simulink model "main"  (R2022b)
settings: Solver=VariableStepAuto  StartTime=0.0  StopTime=inf  RelTol=1e-3
settings Model: Creator=PSSENL  LastModifiedBy=rhdej
settings DebuggingCC: UnderSpecifiedDimensionMsg=warning

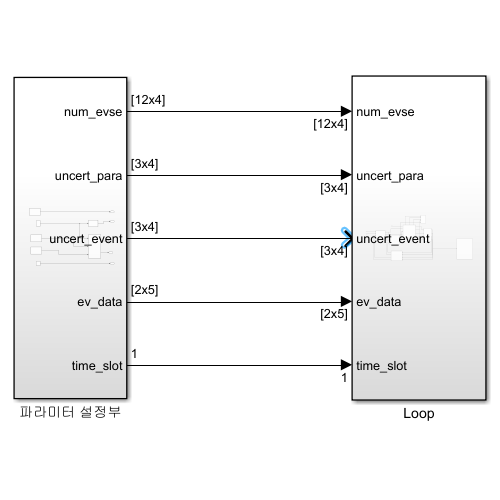
[thumbnail: Simulink's stored preview of the top-level diagram]
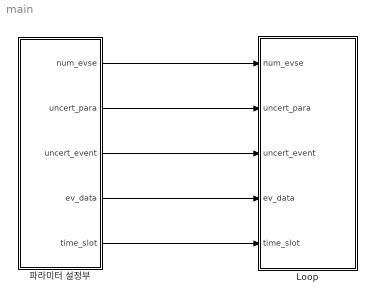
== system main ==
  Loop : Subsystem
  파라미터 설정부 : Subsystem
  wires:
  파라미터 설정부/1(num_evse) -> Loop/1(num_evse)
  파라미터 설정부/4(ev_data) -> Loop/4(ev_data)
  파라미터 설정부/5(time_slot) -> Loop/5(time_slot)
  파라미터 설정부/2(uncert_para) -> Loop/2(uncert_para)
  파라미터 설정부/3(uncert_event) -> Loop/3(uncert_event)

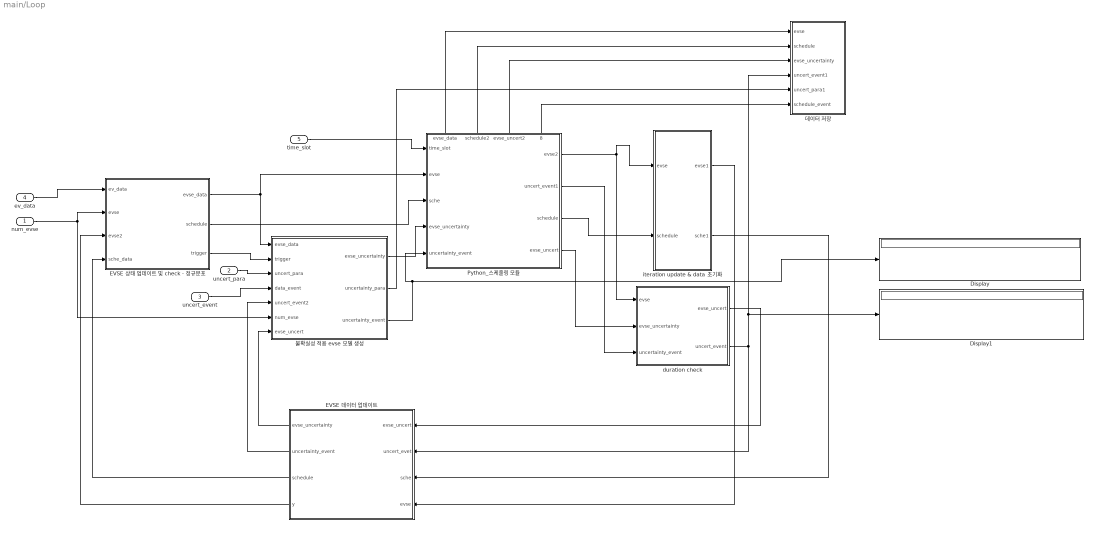
== system main/Loop ==
  num_evse : Inport
  uncert_para : Inport  Port=2
  uncert_event : Inport  Port=3
  ev_data : Inport  Port=4
  time_slot : Inport  Port=5
  Display : Display
  Display1 : Display
  EVSE 데이터 업데이트 : Subsystem
  EVSE 상태 업데이트 및 check - 정규분포 : Subsystem  TreatAsAtomicUnit=on
      settings: MinAlgLoopOccurrences=on
  Python_스케줄링 모듈 : Subsystem  TreatAsAtomicUnit=on
      settings: MinAlgLoopOccurrences=on  PortSchema="{\"entries\":[{\"content\":{\"sides\":[{\"content\":{\"connectorIds\":[\"In1\",\"In2\",\"In3\",\"In4\",\"In5\"]},\"type\":\"ConnectorPlacement.EquallySpacedRectSide\",\"uuid\":\"108a50dd-ff78-47a2-96bb-1485fa352ef4\"},{\"content\":{\"connectorIds\":[\"Out1\",\"Out2\",\"Out3\",\"Out4\"],\"side\":\"RIGHT\"},\"type\":\"ConnectorPlacement.EquallySpacedRectSide\",\"uuid\":\"7c56c117-e709-4297-be3e-b9108604eb1e\"},{\"content\":{\"connectorIds\":[\"Out5\",\"Out6\",\"Out7\",\"Out8\"],\"side\":\"TOP\"},\"type\":\"ConnectorPlacement.EquallySpacedRectSide\",\"uuid\":\"1739f009-047f-4f60-ac68-86188e95dc24\"}]},\"type\":\"ConnectorPlacement.EquallySpacedConnector\",\"uuid\":\"a87990c0-fd82-4870-9496-759f08e65f9c\"}],\"packageUris\":[\"http://schema.mathworks.com/mf0/Connector/R2020b\"],\"version\":\"1.0\"}"
  duration check : MATLAB Function  TreatAsAtomicUnit=on
  iteration update & data 초기화 : MATLAB Function  TreatAsAtomicUnit=on
  데이터 저장 : Subsystem  TreatAsAtomicUnit=on
      settings: MinAlgLoopOccurrences=on
  불확실성 적용 evse 모델 생성 : Subsystem
  wires:
  EVSE 상태 업데이트 및 check - 정규분포/1(evse_data) -> 불확실성 적용 evse 모델 생성/1(evse_data), Python_스케줄링 모듈/2(evse)
  ev_data/1 -> EVSE 상태 업데이트 및 check - 정규분포/1(ev_data)
  iteration update & data 초기화/1(evse1) -> EVSE 데이터 업데이트/4(evse)
  iteration update & data 초기화/2(sche1) -> EVSE 데이터 업데이트/3(sche)
  num_evse/1 -> 불확실성 적용 evse 모델 생성/6(num_evse), EVSE 상태 업데이트 및 check - 정규분포/2(evse)
  EVSE 데이터 업데이트/4(y) -> EVSE 상태 업데이트 및 check - 정규분포/3(evse2)
  EVSE 상태 업데이트 및 check - 정규분포/2(schedule) -> Python_스케줄링 모듈/3(sche)
  Python_스케줄링 모듈/1(evse2) -> iteration update & data 초기화/1(evse), duration check/1(evse)
  Python_스케줄링 모듈/3(schedule) -> iteration update & data 초기화/2(schedule)
  time_slot/1 -> Python_스케줄링 모듈/1(time_slot)
  Python_스케줄링 모듈/5(evse_data) -> 데이터 저장/1(evse)
  Python_스케줄링 모듈/6(schedule2) -> 데이터 저장/2(schedule)
  EVSE 데이터 업데이트/3(schedule) -> EVSE 상태 업데이트 및 check - 정규분포/4(sche_data)
  uncert_para/1 -> 불확실성 적용 evse 모델 생성/3(uncert_para)
  uncert_event/1 -> 불확실성 적용 evse 모델 생성/4(data_event)
  EVSE 상태 업데이트 및 check - 정규분포/3(trigger) -> 불확실성 적용 evse 모델 생성/2(trigger)
  불확실성 적용 evse 모델 생성/1(evse_uncertainty) -> Python_스케줄링 모듈/4(evse_uncertainty)
  불확실성 적용 evse 모델 생성/3(uncertainty_event) -> Python_스케줄링 모듈/5(uncertainty_event), Display/1
  duration check/2(uncert_event) -> EVSE 데이터 업데이트/2(uncert_evet), 데이터 저장/4(uncert_event1), Display1/1
  duration check/1(evse_uncert) -> EVSE 데이터 업데이트/1(evse_uncert)
  Python_스케줄링 모듈/4(evse_uncert) -> duration check/2(evse_uncertainty)
  EVSE 데이터 업데이트/1(evse_uncertainty) -> 불확실성 적용 evse 모델 생성/7(evse_uncert)
  Python_스케줄링 모듈/7(evse_uncert2) -> 데이터 저장/3(evse_uncertainty)
  Python_스케줄링 모듈/2(uncert_event1) -> duration check/3(uncertainty_event)
  불확실성 적용 evse 모델 생성/2(uncertainty_para) -> 데이터 저장/5(uncert_para1)
  EVSE 데이터 업데이트/2(uncertainty_event) -> 불확실성 적용 evse 모델 생성/5(uncert_event2)
  Python_스케줄링 모듈/8(schedule_event) -> 데이터 저장/6(schedule_event)

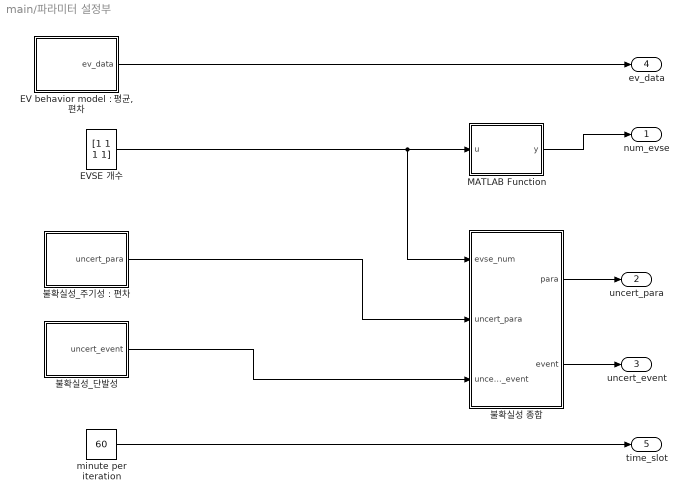
== system main/파라미터 설정부 ==
  "EV behavior model : 평균, 편차" : Subsystem
  EVSE 개수 : Constant  Value=[1 1 1 1]
  MATLAB Function : MATLAB Function  TreatAsAtomicUnit=on
  minute per iteration : Constant  Value=60
  불확실성 종합 : MATLAB Function  TreatAsAtomicUnit=on
  불확실성_단발성 : Subsystem
  "불확실성_주기성 : 편차" : Subsystem
  num_evse : Outport
  uncert_para : Outport  Port=2
  uncert_event : Outport  Port=3
  ev_data : Outport  Port=4
  time_slot : Outport  Port=5
  wires:
  EVSE 개수/1 -> 불확실성 종합/1(evse_num), MATLAB Function/1(u)
  MATLAB Function/1(y) -> num_evse/1
  "EV behavior model : 평균, 편차"/1(ev_data) -> ev_data/1
  minute per iteration/1 -> time_slot/1
  불확실성_단발성/1(uncert_event) -> 불확실성 종합/3(uncert_event)
  "불확실성_주기성 : 편차"/1(uncert_para) -> 불확실성 종합/2(uncert_para)
  불확실성 종합/1(para) -> uncert_para/1
  불확실성 종합/2(event) -> uncert_event/1

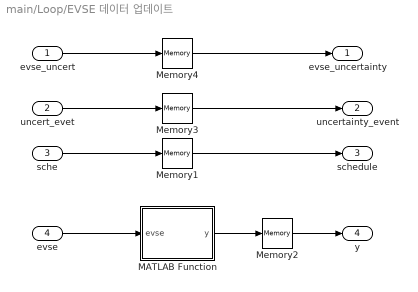
== system main/Loop/EVSE 데이터 업데이트 ==
  evse_uncert : Inport
  uncert_evet : Inport  Port=2
  sche : Inport  Port=3
  evse : Inport  Port=4
  MATLAB Function : MATLAB Function  TreatAsAtomicUnit=on
  Memory{1..4} (4 alike) : Memory
  evse_uncertainty : Outport
  uncertainty_event : Outport  Port=2
  schedule : Outport  Port=3
  y : Outport  Port=4
  wires:
  evse/1 -> MATLAB Function/1(evse)
  MATLAB Function/1(y) -> Memory2/1
  sche/1 -> Memory1/1
  Memory1/1 -> schedule/1
  Memory2/1 -> y/1
  evse_uncert/1 -> Memory4/1
  uncert_evet/1 -> Memory3/1
  Memory3/1 -> uncertainty_event/1
  Memory4/1 -> evse_uncertainty/1

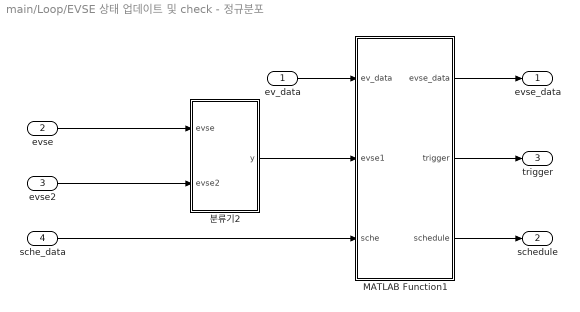
== system main/Loop/EVSE 상태 업데이트 및 check - 정규분포 ==
  ev_data : Inport
  evse : Inport  Port=2
  evse2 : Inport  Port=3
  sche_data : Inport  Port=4
  MATLAB Function1 : MATLAB Function  TreatAsAtomicUnit=on
  분류기2 : MATLAB Function  TreatAsAtomicUnit=on
  evse_data : Outport
  schedule : Outport  Port=2
  trigger : Outport  Port=3
  wires:
  MATLAB Function1/1(evse_data) -> evse_data/1
  ev_data/1 -> MATLAB Function1/1(ev_data)
  evse/1 -> 분류기2/1(evse)
  분류기2/1(y) -> MATLAB Function1/2(evse1)
  evse2/1 -> 분류기2/2(evse2)
  sche_data/1 -> MATLAB Function1/3(sche)
  MATLAB Function1/3(schedule) -> schedule/1
  MATLAB Function1/2(trigger) -> trigger/1

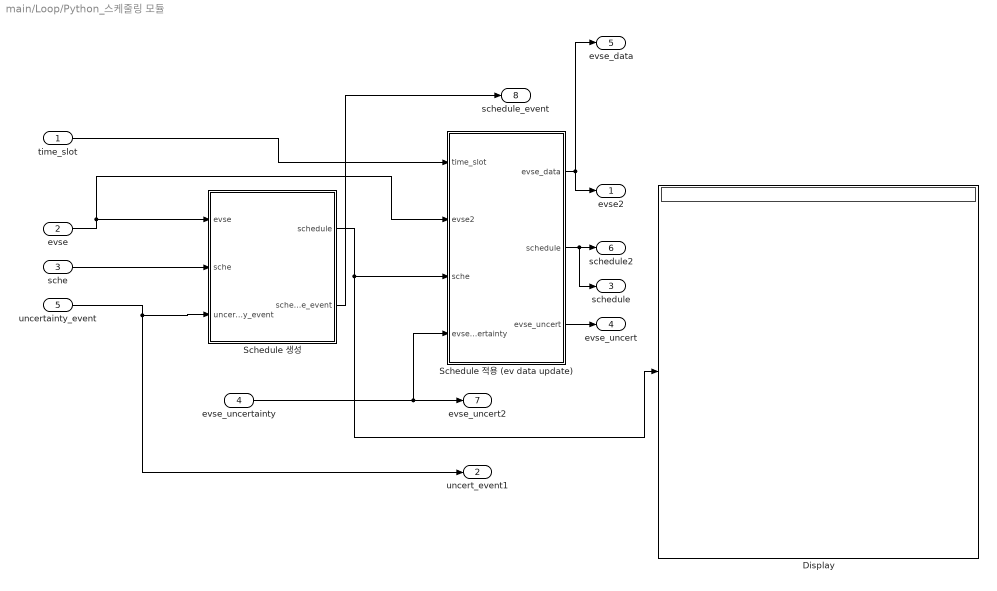
== system main/Loop/Python_스케줄링 모듈 ==
  time_slot : Inport
  evse : Inport  Port=2
  sche : Inport  Port=3
  evse_uncertainty : Inport  Port=4
  uncertainty_event : Inport  Port=5
  Display : Display
  Schedule 생성 : MATLAB Function  TreatAsAtomicUnit=on
  Schedule 적용 (ev data update) : MATLAB Function  TreatAsAtomicUnit=on
  evse2 : Outport
  uncert_event1 : Outport  Port=2
  schedule : Outport  Port=3
  evse_uncert : Outport  Port=4
  evse_data : Outport  Port=5
  schedule2 : Outport  Port=6
  evse_uncert2 : Outport  Port=7
  schedule_event : Outport  Port=8
  wires:
  Schedule 생성/1(schedule) -> Display/1, Schedule 적용 (ev data update)/3(sche)
  sche/1 -> Schedule 생성/2(sche)
  evse/1 -> Schedule 적용 (ev data update)/2(evse2), Schedule 생성/1(evse)
  Schedule 적용 (ev data update)/1(evse_data) -> evse2/1, evse_data/1
  Schedule 적용 (ev data update)/2(schedule) -> schedule/1, schedule2/1
  time_slot/1 -> Schedule 적용 (ev data update)/1(time_slot)
  evse_uncertainty/1 -> Schedule 적용 (ev data update)/4(evse_uncertainty), evse_uncert2/1
  uncertainty_event/1 -> Schedule 생성/3(uncertainty_event), uncert_event1/1
  Schedule 적용 (ev data update)/3(evse_uncert) -> evse_uncert/1
  Schedule 생성/2(schedule_event) -> schedule_event/1

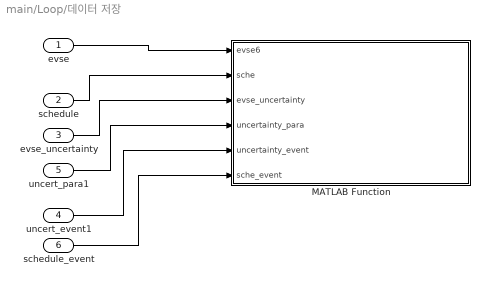
== system main/Loop/데이터 저장 ==
  evse : Inport
  schedule : Inport  Port=2
  evse_uncertainty : Inport  Port=3
  uncert_event1 : Inport  Port=4
  uncert_para1 : Inport  Port=5
  schedule_event : Inport  Port=6
  MATLAB Function : MATLAB Function  TreatAsAtomicUnit=on
  wires:
  evse/1 -> MATLAB Function/1(evse6)
  schedule/1 -> MATLAB Function/2(sche)
  evse_uncertainty/1 -> MATLAB Function/3(evse_uncertainty)
  uncert_para1/1 -> MATLAB Function/4(uncertainty_para)
  uncert_event1/1 -> MATLAB Function/5(uncertainty_event)
  schedule_event/1 -> MATLAB Function/6(sche_event)

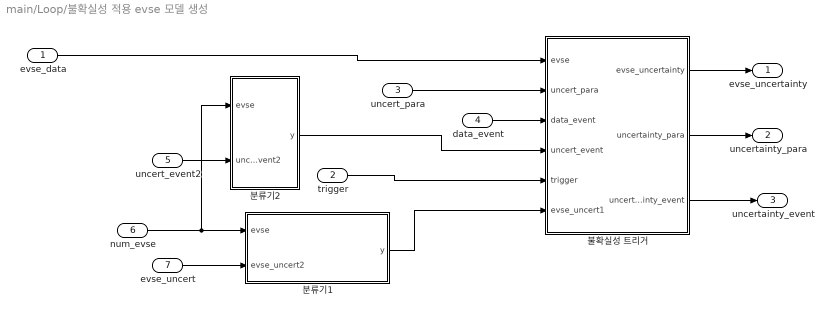
== system main/Loop/불확실성 적용 evse 모델 생성 ==
  evse_data : Inport
  trigger : Inport  Port=2
  uncert_para : Inport  Port=3
  data_event : Inport  Port=4
  uncert_event2 : Inport  Port=5
  num_evse : Inport  Port=6
  evse_uncert : Inport  Port=7
  분류기1 : MATLAB Function  TreatAsAtomicUnit=on
  분류기2 : MATLAB Function  TreatAsAtomicUnit=on
  불확실성 트리거 : MATLAB Function  TreatAsAtomicUnit=on
  evse_uncertainty : Outport
  uncertainty_para : Outport  Port=2
  uncertainty_event : Outport  Port=3
  wires:
  uncert_para/1 -> 불확실성 트리거/2(uncert_para)
  data_event/1 -> 불확실성 트리거/3(data_event)
  trigger/1 -> 불확실성 트리거/5(trigger)
  불확실성 트리거/1(evse_uncertainty) -> evse_uncertainty/1
  불확실성 트리거/2(uncertainty_para) -> uncertainty_para/1
  불확실성 트리거/3(uncertainty_event) -> uncertainty_event/1
  evse_uncert/1 -> 분류기1/2(evse_uncert2)
  uncert_event2/1 -> 분류기2/2(uncert_event2)
  분류기2/1(y) -> 불확실성 트리거/4(uncert_event)
  분류기1/1(y) -> 불확실성 트리거/6(evse_uncert1)
  num_evse/1 -> 분류기2/1(evse), 분류기1/1(evse)
  evse_data/1 -> 불확실성 트리거/1(evse)

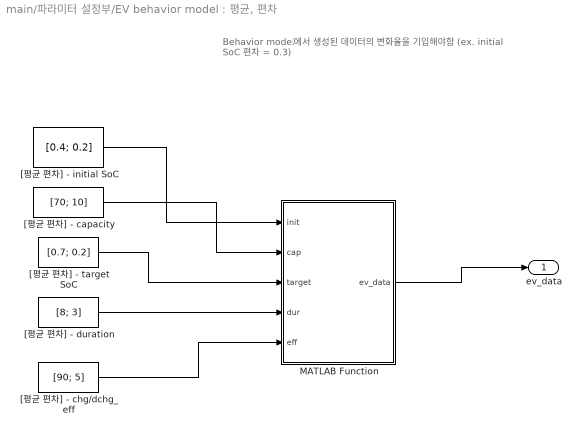
== system main/파라미터 설정부/EV behavior model : 평균, 편차 ==
  note: Behavior model에서 생성된 데이터의 변화율을 기입해야함
      | (ex. initial SoC 편차 = 0.3)
  MATLAB Function : MATLAB Function  TreatAsAtomicUnit=on
  "[평균 편차] - capacity" : Constant  Value=[70; 10]
  "[평균 편차] - chg/dchg_eff" : Constant  Value=[90; 5]
  "[평균 편차] - duration" : Constant  Value=[8; 3]
  "[평균 편차] - initial SoC" : Constant  Value=[0.4; 0.2]
  "[평균 편차] - target SoC" : Constant  Value=[0.7; 0.2]
  ev_data : Outport
  wires:
  "[평균 편차] - initial SoC"/1 -> MATLAB Function/1(init)
  "[평균 편차] - capacity"/1 -> MATLAB Function/2(cap)
  "[평균 편차] - target SoC"/1 -> MATLAB Function/3(target)
  "[평균 편차] - duration"/1 -> MATLAB Function/4(dur)
  MATLAB Function/1(ev_data) -> ev_data/1
  "[평균 편차] - chg/dchg_eff"/1 -> MATLAB Function/5(eff)

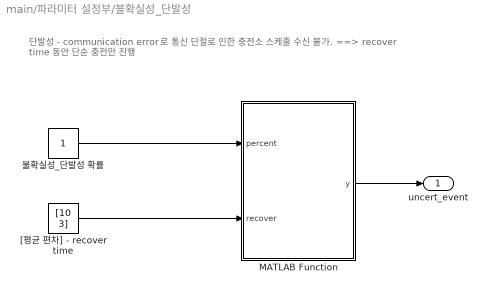
== system main/파라미터 설정부/불확실성_단발성 ==
  note: 단발성 - communication error 로 통신 단절로 인한 충전소 스케줄 수신 불가.
      | ==> recover time 동안 단순 충전만 진행
  MATLAB Function : MATLAB Function  TreatAsAtomicUnit=on
  "[평균 편차] - recover time" : Constant  Value=[10 3]
  불확실성_단발성 확률 : Constant
  uncert_event : Outport
  wires:
  MATLAB Function/1(y) -> uncert_event/1
  "[평균 편차] - recover time"/1 -> MATLAB Function/2(recover)
  불확실성_단발성 확률/1 -> MATLAB Function/1(percent)

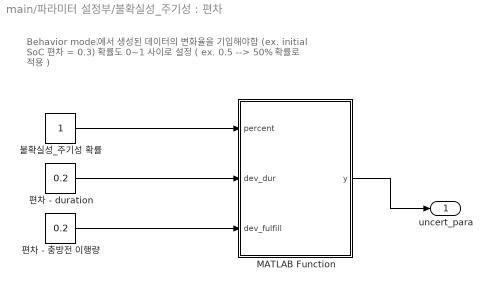
== system main/파라미터 설정부/불확실성_주기성 : 편차 ==
  note: Behavior model에서 생성된 데이터의 변화율을 기입해야함
      | (ex. initial SoC 편차 = 0.3)
      | 확률도 0~1 사이로 설정 ( ex. 0.5 --> 50% 확률로 적용 )
  MATLAB Function : MATLAB Function  TreatAsAtomicUnit=on
  불확실성_주기성 확률 : Constant
  편차 - duration : Constant  Value=0.2
  편차 - 충방전 이행량 : Constant  Value=0.2
  uncert_para : Outport
  wires:
  편차 - duration/1 -> MATLAB Function/2(dev_dur)
  편차 - 충방전 이행량/1 -> MATLAB Function/3(dev_fulfill)
  MATLAB Function/1(y) -> uncert_para/1
  불확실성_주기성 확률/1 -> MATLAB Function/1(percent)

== matlab function main/Loop/Python_스케줄링 모듈/Schedule 생성 ==
  data: evse input; schedule output; sche input; uncertainty_event input; schedule_event output
% event - 1: iteration 2: state 3: recover

function [schedule,schedule_event] = fcn(evse, sche, uncertainty_event)
coder.extrinsic("writematrix")
coder.extrinsic("readmatrix")

sche_sample = readmatrix("input/sample schedule.csv");
evse_num = size(evse,2);
sche_data1 = zeros(25,evse_num);
sche_data2 = zeros(25,evse_num);
schedule = zeros(25,evse_num);
schedule_event = zeros(25,evse_num);

% EVSE 상태에 따른 스케줄 생성
for i = 1:evse_num
    if (evse(1,i) == 1) && (evse(3,i) ~= 0) % state check
        for j = 1 : 24
            sche_data1(j,i) = sche_sample(j,i); % schedule 생성
            sche_data2(j,i) = sche_sample(j,i); % schedule 생성
            sche_data1(25,i) = 1;
            sche_data2(25,i) = 1;

            % event - communication error --> dumb charging
            if (uncertainty_event(1,i) ~= 0) && (uncertainty_event(2,i) == 1) && (uncertainty_event(3,i) ~= 0)
                sche_data2(j,i) = 8;
            end
        end
    end
end

% schedule iteration check
if size(sche,1) == 25
    for i = 1:evse_num
        iter_sche = sche(25,i);
        if iter_sche == 0
            sche_data1(25,i) = 1;
        else
            sche_data1(25,i) = sche(25,i);
        end
        if evse(1,i) == 0
            sche_data1(25,i) = 0;
        end
    end
end

schedule = sche_data1;
schedule_event = sche_data2;

== matlab function main/파라미터 설정부/불확실성_단발성/MATLAB Function ==
  data: y output; percent input; recover input
% 1: percent 2:recover mean 3: recover deviation
function y = fcn(percent, recover)

col = size(percent,1)+size(recover,1);
y = zeros(1,col);
y = [percent transpose(recover)];
end

== matlab function main/Loop/불확실성 적용 evse 모델 생성/불확실성 트리거 ==
  data: evse input; evse_uncertainty output; uncert_para input; data_event input; uncert_event input; trigger input; uncertainty_para output; uncertainty_event output; evse_uncert1 input
% para - 1: percent 2: dur 3: fulfill
% event - 1: percent 2:recover mean 3: recover deviation

% 1 : state, 2:iteration 3: cap, 4: init, 5: target, 6: min, 7:max
% 8 : dur, 9: Pmin, 10: Pmax, 11 : chg_eff, 12: dchg_eff

function [evse_uncertainty,uncertainty_para, uncertainty_event] = fcn(evse, uncert_para, data_event, uncert_event, trigger, evse_uncert1)
coder.extrinsic("binornd", "randn", "rng")
rng shuffle

err_dur = zeros(1,size(evse,2)); % duration 오차율
err_eff = zeros(1,size(evse,2)); % efficiency 오차율
evse_uncert = zeros(12,size(evse,2)); % evse_data uncertainty version
uncert_event1 = zeros(3,size(evse,2));

uncert_para1 = zeros(3,size(evse,2));

state_para = zeros(1,size(evse,2)); % 주기성 상태

%% 트리거 변수에 따른 스케줄링 불확실성 적용버전 생성
for i = 1:size(evse,2)
    % parameter uncertainty generation
    % EV model generation check
    if trigger(1,i) == 1
        % uncertainty generation
        state_para(1,i) = binornd(1,uncert_para(1,i));
        % uncertainty generation check
        if state_para(1,i) == 1
            %duration
            dur = 0;
            dur = randn * uncert_para(2,i);

            % 무조건 음수로
            if dur > 0
                dur = -dur;
            end
            err_dur(1,i) = dur;

            % efficiency
            eff = 0;
            eff = randn * uncert_para(3,i);

            % 무조건 음수로
            if eff > 0
                eff = -eff;
            end
            err_eff(1,i) = eff;

            % EVSE 적용
            evse_uncert(:,i) = evse(:,i);
            evse_uncert(8,i) = round(evse_uncert(8,i) * (1 + err_dur(1,i))); % duration
            evse_uncert(11,i) = round(evse_uncert(11,i) * (1 + err_eff(1,i))); % chg_eff
            evse_uncert(12,i) = evse_uncert(11,i);
        else
            evse_uncert(:,i) = -1; % trigger 됐으나, 불확실성 모델이 생성 안된 case
        end

    elseif (trigger(1,i) ~= 1)
        for j = 1:12
            evse_uncert(j,i) = evse_uncert1(j,i); % trigger 되지 않은 case : 이전 불확실성 데이터 저장
        end
    end
    uncert_para1(1,i) = state_para(1,i);
    uncert_para1(2,i) = err_dur(1,i);
    uncert_para1(3,i) = err_eff(1,i);
    trigger(1,i) = 0;

%% event ucnertainty generation
    if size(uncert_event,1) ~= 1
        if (uncert_event(2,i) == 0)
            event_state = 0;
            event_state = binornd(1,data_event(1,i));
            uncert_event1(2,i) = event_state;
            % event state check
            if uncert_event1(2,i) == 1
                recover_dev = 0;
                recover_dev = data_event(3,i) * randn;
                data_recover = 0;
                data_recover = data_event(2,i) + recover_dev;
                uncert_event1(3,i) = round(data_recover);
            end
            uncert_event1(1,i) = uncert_event(1,i) + 1;
        else
            uncert_event1(:,i) = uncert_event(:,i);
        end
    end
end


% event_parameter - 1: probability 2: recover mean 3: recover devi
% event - 1: iteration 2: state 3: recover

uncertainty_para = uncert_para1;
uncertainty_event = uncert_event1;
evse_uncertainty = zeros(12,size(evse,2));
evse_uncertainty = evse_uncert;

== matlab function main/Loop/불확실성 적용 evse 모델 생성/분류기2 ==
  data: evse input; y output; uncert_event2 input
% event - 1: iteration 2: state 3: recover_time

function y = fcn(evse, uncert_event2)
evse_num = size(evse,2);

event_state = zeros(3,evse_num);

% evse 데이터 분류
if size(event_state) == size(uncert_event2)
    event_state = uncert_event2;
end

y = event_state;

== matlab function main/Loop/EVSE 상태 업데이트 및 check - 정규분포/분류기2 ==
  data: y output; evse input; evse2 input
% 1 : state, 2:iteration 3: cap, 4: init, 5: target, 6: min, 7:max
% 8 : dur, 9: Pmin, 10: Pmax, 11 : chg_eff, 12: dchg_eff

function y = fcn(evse, evse2)
coder.extrinsic("delete")

evse_data = zeros(size(evse));
evse_data = evse;

% evse 데이터 분류
if size(evse2,1) == 12
    evse_data = evse2;
end

% 이전 시뮬레이션 결과 삭제    
for i = 1:size(evse,2)
    if evse_data(2,i) == 0
        txt1 = sprintf('result/normal/evse_%d.csv',int8(i));
        txt2 = sprintf('result/normal/schedule_%d.csv',int8(i));
        txt3 = sprintf('result/state/parameter_%d.csv',int8(i));
        txt4 = sprintf('result/state/event_%d.csv',int8(i));
        txt5 = sprintf('result/uncertainty/evse_%d.csv',int8(i));
        txt6 = sprintf('result/uncertainty/schedule_%d.csv',int8(i));
        delete(txt1);
        delete(txt2);
        delete(txt3);
        delete(txt4);
        delete(txt5);
        delete(txt6);
    end
end

y = zeros(size(evse));
y = evse_data;

== matlab function main/Loop/iteration update & data 초기화 ==
  data: evse input; evse1 output; schedule input; sche1 output
% 1 : state, 2:iteration 3: cap, 4: init, 5: target, 6: min, 7:max
% 8 : dur, 9: Pmin, 10: Pmax, 11 : chg_eff, 12: dchg_eff

% 1: init 2:cap 3:target 4:dur 5:eff

function [evse1,sche1] = fcn(evse ,schedule)
state1 = zeros(size(evse)); % evse의 ev 모델
evse1 = zeros(12,size(evse,2)); % evse output
sche1 = zeros(25,size(schedule,2)); % evse별 스케줄
sche_data = zeros(25,size(schedule,2));
sche_data = schedule;

iter_evse = 0; % evse iteration
iter_sche = 0; % schedule iteration

state1 = evse; % input

% evse iteration update
for i = 1:size(state1,2)
    if (state1(8,i) == 0)
        iter_evse = state1(2,i);
        state1(:,i) = 0;
        state1(2,i) = iter_evse;
        for j = 1:25
            sche_data(j,i) = 0;
        end
    end
end

% schedule iteration update
for i = 1:size(state1,2)
    if (state1(1,i) == 1)
        iter_sche = sche_data(25,i);
        iter_sche = iter_sche + 1;
        sche_data(25,i) = iter_sche;
    end
end


%schedule matching with evse state
for i = 1:size(state1,2)
    if (25 == 25) && ((state1(1,i) == 0) || (state1(8,i) == 0))
        sche_data(25,i) = 0;
    end
end


evse1 = state1;
sche1 = sche_data;

== matlab function main/Loop/데이터 저장/MATLAB Function ==
  data: evse6 input; sche input; evse_uncertainty input; uncertainty_para input; uncertainty_event input; sche_event input
% 1 : state, 2:iteration 3: cap, 4: init, 5: target, 6: min, 7:max
% 8 : dur, 9: Pmin, 10: Pmax, 11 : chg_eff, 12: dchg_eff

function fcn(evse6, sche, evse_uncertainty, uncertainty_para, uncertainty_event, sche_event)
coder.extrinsic("writematrix")
coder.extrinsic("readmatrix")
coder.extrinsic("int8")
coder.extrinsic("exist")

evse_num = size(evse6,2);
iter_sche = 0;
iter_sche2 = 0;
a = 0;
b = 0;
c = 0;
d = 0;
e = 0;
f = 0;
row_num = 0;
row_num2 = 0;
row_num_sche = 0;
row_num_sche2 = 0;
row_num_event = 0;
row_num_para = 0;


for i = 1:evse_num
    % evse 저장
    txt1 = sprintf('result/normal/evse_%d.csv',int8(i));
    a = exist(txt1);
    if a == 0
        ev_data = zeros(1,size(evse6,1));
        writematrix(ev_data,txt1);
        data_evse1 = readmatrix(txt1);
        data_evse2 = zeros(row_num + 1,12);
        data_evse2 = vertcat(data_evse1, transpose(evse6(:,i)));
        writematrix(data_evse2,txt1);
    else
        data_evse1 = readmatrix(txt1);
        row_num = size(data_evse1,1);
        data_evse2 = zeros(row_num + 1,12);
        data_evse2 = vertcat(data_evse1, transpose(evse6(:,i)));
        writematrix(data_evse2,txt1);
    end


    % schedule 저장
    txt2 = sprintf('result/normal/schedule_%d.csv',int8(i));
    b = exist(txt2);
    iter_sche = sche(25,i);
    if b == 0
        for j = 1 : size(sche,1)
            data_sche = zeros(1,size(sche,1));
            data_sche3 = zeros(2,size(sche,1));
            writematrix(data_sche3,txt2);
            data_sche(1,1:iter_sche) = sche(1:iter_sche,i);
            data_sche2 = zeros(row_num_sche+1,size(sche,1));
            data_sche3 = vertcat(data_sche3,data_sche);
            writematrix(data_sche,txt2);
        end
    else
        data_sche5 = readmatrix(txt2);
        row_num_sche = size(data_sche5,1);
        data_sche3 = zeros(row_num_sche + 1,size(sche,1));
        data_sche4 = zeros(1,size(sche,1));
        for j = 1:size(sche,1)
            data_sche4(1,1:iter_sche) = sche(1:iter_sche,i);
            if j == 25
                data_sche4(1,j) = sche(j,i);
            end
        end
        data_sche3 = vertcat(data_sche5,data_sche4);
        writematrix(data_sche3,txt2);
    end


    % % uncertainty_para 저장


    txt3 = sprintf('result/state/parameter_%d.csv',int8(i));
    c = exist(txt3);
    if c == 0
        para_data = zeros(1,size(uncertainty_para,1));
        writematrix(para_data,txt3);
        para_data1 = readmatrix(txt3);
        para_data2 = zeros(row_num_para + 1,size(uncertainty_para,1));
        para_data2 = vertcat(para_data1, transpose(uncertainty_para(:,i)));
        writematrix(para_data2,txt3);
    else
        para_data1 = readmatrix(txt3);
        row_num_para = size(para_data1,1);
        para_data2 = zeros(row_num_para + 1,size(uncertainty_para,1));
        para_data2 = vertcat(para_data1, transpose(uncertainty_para(:,i)));
        writematrix(para_data2,txt3);
    end


    % % uncertainty_event 저장

    txt4 = sprintf('result/state/event_%d.csv',int8(i));
    d = exist(txt4);
    if d == 0
        event_data = zeros(1,size(uncertainty_event,1));
        writematrix(event_data,txt4);
        event_data1 = readmatrix(txt4);
        event_data2 = zeros(row_num_event + 1,size(uncertainty_event,1));
        event_data2 = vertcat(event_data1, transpose(uncertainty_event(:,i)));
        writematrix(event_data2,txt4);
    else
        event_data1 = readmatrix(txt4);
        row_num_event = size(event_data1,1);
        event_data2 = zeros(row_num_event + 1,size(uncertainty_event,1));
        event_data2 = vertcat(event_data1, transpose(uncertainty_event(:,i)));
        writematrix(event_data2,txt4);
    end


    % uncertainty_evse 저장

    txt5 = sprintf('result/uncertainty/evse_%d.csv',int8(i));
    e = exist(txt5);
    if e == 0
        ev_data2 = zeros(1,size(evse_uncertainty,1));
        writematrix(ev_data2,txt5);
        data_evse_un1 = readmatrix(txt5);
        data_evse_un2 = zeros(row_num2 + 1,12);
        data_evse_un2 = vertcat(data_evse_un1, transpose(evse_uncertainty(:,i)));
        writematrix(data_evse_un2,txt5);
    else
        data_evse_un1 = readmatrix(txt5);
        row_num2 = size(data_evse_un1,1);
        data_evse_un2 = zeros(row_num2 + 1,12);
        data_evse_un2 = vertcat(data_evse_un1, transpose(evse_uncertainty(:,i)));
        writematrix(data_evse_un2,txt5);
    end

    % schedule_event 저장
    txt6 = sprintf('result/uncertainty/schedule_%d.csv',int8(i));
    f = exist(txt6);
    iter_sche2 = sche_event(25,i);
    if f == 0
        for j = 1 : size(sche_event,1)
            data_sche_event = zeros(1,size(sche_event,1));
            data_sche3_event = zeros(2,size(sche_event,1));
            writematrix(data_sche3_event,txt6);
            data_sche_event(1,1:iter_sche2) = sche_event(1:iter_sche2,i);
            data_sche2_event = zeros(row_num_sche2+1,size(sche_event,1));
            data_sche3_event = vertcat(data_sche3_event,data_sche_event);
            writematrix(data_sche_event,txt6);
        end
    else
        data_sche5_event = readmatrix(txt6);
        row_num_sche2 = size(data_sche5_event,1);
        data_sche3_event = zeros(row_num_sche2 + 1,size(sche_event,1));
        data_sche4_event = zeros(1,size(sche_event,1));
        for j = 1:size(sche_event,1)
            data_sche4_event(1,1:iter_sche2) = sche_event(1:iter_sche2,i);
            if j == 25
                data_sche4_event(1,j) = sche_event(j,i);
            end
        end
        data_sche3_event = vertcat(data_sche5_event,data_sche4_event);
        writematrix(data_sche3_event,txt6);
    end
end

== matlab function main/Loop/불확실성 적용 evse 모델 생성/분류기1 ==
  data: evse input; y output; evse_uncert2 input
% 1 : state, 2:iteration 3: cap, 4: init, 5: target, 6: min, 7:max
% 8 : dur, 9: Pmin, 10: Pmax, 11 : chg_eff, 12: dchg_eff

function y = fcn(evse, evse_uncert2)
coder.extrinsic("delete")

evse_uncert = zeros(12,size(evse,2));

% evse 데이터 분류
if size(evse_uncert2) == size(evse_uncert)
    evse_uncert = evse_uncert2;
end

y = zeros(12,size(evse,2));
y = evse_uncert;

== matlab function main/파라미터 설정부/불확실성 종합 ==
  settings: updateMethod=DISCRETE
  data: para output [1..100]; evse_num input; uncert_para input; uncert_event input; event output
% para - 1: percent 2: dur 3: fulfill
% event - 1: percent 2:recover mean 3: recover deviation

function [para,event] = fcn(evse_num, uncert_para, uncert_event)

col = size(evse_num,1);
row_para = size(uncert_para,2);
row_event = size(uncert_event,2);

para1 = zeros(row_para,col);
event1 = zeros(row_event,col);

for i = 1:col
    para1(:,i) = uncert_para(1,:);
    event1(:,i) = uncert_event(1,:);
end

para = para1;
event = event1;

== matlab function main/파라미터 설정부/MATLAB Function ==
  data: u input; y output [1..100]
function y = fcn(u)
% 1 : state, 2:iteration 3: cap, 4: init, 5: target, 6: min, 7:max
% 8 : dur, 9: Pmin, 10: Pmax, 11 : chg_eff, 12: dchg_eff

num_cols = size(u, 1);
y = zeros(12, num_cols);
end

== matlab function main/파라미터 설정부/불확실성_주기성 : 편차/MATLAB Function ==
  data: percent input; y output; dev_dur input; dev_fulfill input
% 1: percent 2:dur 3:fulfill
function y = fcn(percent, dev_dur, dev_fulfill)

col = size(dev_dur,1)+size(dev_fulfill,1)+size(percent,1);
y = zeros(1,col);
y = [percent dev_dur dev_fulfill];
end

== matlab function main/Loop/EVSE 데이터 업데이트/MATLAB Function ==
  settings: updateMethod=DISCRETE
  data: evse input; y output
function y= fcn(evse)
coder.extrinsic("round","binornd","rng")

rng shuffle

% 운용 가능 플러그 개수 확인하기
idx = find(evse(1,:)==0);
empty_num = size(find(evse(1,:) == 0),2);

% 운용 가능 플러그 개수만큼 분포 발생하기
if sum(empty_num) ~= 0
   for i = 1:empty_num
       evse(1,idx(i)) = binornd(1,0.5);
   end
end

y = evse;

== matlab function main/파라미터 설정부/EV behavior model : 평균, 편차/MATLAB Function ==
  data: init input; ev_data output; cap input; target input; dur input; eff input
% 1: init 2:cap 3:target 4:dur 5:eff
function ev_data = fcn(init, cap, target, dur, eff)
ev_data = [init cap target dur eff];

end

== matlab function main/Loop/EVSE 상태 업데이트 및 check - 정규분포/MATLAB Function1 ==
  data: evse_data output; trigger output; ev_data input; evse1 input; sche input; schedule output
% 1 : state, 2:iteration 3: cap, 4: init, 5: target, 6: min, 7:max
% 8 : dur, 9: Pmin, 10: Pmax, 11 : chg_eff, 12: dchg_eff

% 1: init 2:cap 3:target 4:dur 5:eff

function [evse_data, trigger, schedule] = fcn(ev_data, evse1, sche)
coder.extrinsic('round')
coder.extrinsic('rng')
coder.extrinsic('randn')

rng('shuffle');

state = zeros(12,size(evse1,2)); % evse data
state = evse1;
trigger1 = zeros(1,size(evse1,2));
trigger = zeros(1,size(evse1,2));

%% evse 상태에 따라 정규분포로 데이터 생성
for i = 1:size(state,2)
    if (state(1,i) == 1) && (state(3,i) == 0)
        cap = 0;
        cap = ev_data(2,2)*randn;
        state(3,i) = round(ev_data(1,2) + cap,1);%capacity

        init = 0;
        init = ev_data(2,1)*randn;
        state(4,i) = round(ev_data(1,1) + init,1); % initial SoC

        target = 0;
        target = ev_data(2,3)*randn;
        state(5,i) = round(ev_data(1,3) + target,2); % target SoC
        state(6,i) = 0.05; % min
        state(7,i) = 0.95; % max
        
        dur = 0;
        dur = ev_data(2,4)*randn;
        state(8,i) = round(ev_data(1,4)+dur); % duration
        state(9,i) = -5; %Pmin
        state(10,i) = 11; %Pmax

        eff = 0;
        eff = ev_data(2,5)*randn;
        state(11,i) = round(ev_data(1,5)+eff); %chg_eff
        state(12,i) = state(11,i); %dchg_eff

        % SoC boundary
        if (state(4,i) < 0) || (state(4,i) > 0.6)
            state(4,i) = 0.2;
        end

        if (state(5,i) >= 1)
            state(5,i) = 0.8;
        end

        %duration minus
        if state(8,i) <= 0
            state(8,i) = 2;
        end

        if state(11,i) >= 100
            state(11,i) = 99;
        end

        state(12,i) = state(11,i); %dchg_eff
        trigger1(1,i) = 1;
    end
end
schedule = zeros(25,size(sche,2));
evse_data = zeros(size(evse1));

trigger = trigger1;
schedule = sche;
evse_data = state;

== matlab function main/Loop/duration check ==
  data: evse input; evse_uncertainty input; uncertainty_event input; evse_uncert output; uncert_event output
% 1 : state, 2:iteration 3: cap, 4: init, 5: target, 6: min, 7:max
% 8 : dur, 9: Pmin, 10: Pmax, 11 : chg_eff, 12: dchg_eff

% 1: init 2:cap 3:target 4:dur 5:eff

function [evse_uncert, uncert_event] = fcn(evse, evse_uncertainty, uncertainty_event)
state = zeros(12,size(evse,2));
state2 = zeros(3,size(evse,2));
evse_uncert = zeros(12,size(evse,2));
uncert_event = zeros(3,size(evse,2));
iter_para = 0; % evse iteration

%% 불확실성 duration check

% para uncertainty update ( evse )
 % iteration
 if size(evse_uncertainty,1) ~= 1
     state = evse_uncertainty;
     for i = 1:size(evse,2)
         if (state(8,i) == 0)
             iter_para = state(2,i);
             state(:,i) = 0;
             state(2,i) = iter_para;
         end
     end
 end
 % event uncertainty update
 if size(uncertainty_event,1) ~= 1
     state2 = uncertainty_event;
     for i = 1:size(evse,2)
         if (state2(2,i) ~= 0) && (state2(3,i) ~= 0)
         state2(1,i) = state2(1,i) + 1; % iteration update
         state2(3,i) = state2(3,i) - 1; % recover time update
            if state2(3,i) == 0
                iter_event = 0;
                iter_event = state2(1,i);
                state2(:,i) = 0;
                state2(1,i) = iter_event;
            end
         end
     end
 end
 % recover_time update
evse_uncert = state;
uncert_event = state2;

== matlab function main/Loop/Python_스케줄링 모듈/Schedule 적용 (ev data update) ==
  data: time_slot input; evse2 input; evse_data output; sche input; schedule output; evse_uncertainty input; evse_uncert output
% 1 : state, 2:iteration 3: cap, 4: init, 5: target, 6: min, 7:max
% 8 : dur, 9: Pmin, 10: Pmax, 11 : chg_eff, 12: dchg_eff

% 1: init 2:cap 3:target 4:dur 5:eff
function [evse_data,schedule, evse_uncert] = fcn(time_slot, evse2, sche, evse_uncertainty)
coder.extrinsic('round')
coder.extrinsic('rng')
coder.extrinsic('randn')

rng('shuffle');

state = zeros(12,size(evse2,2)); % evse data
state = evse2;

state2 = zeros(12,size(evse2,2)); % evse uncertainty data
state2 = evse_uncertainty;

iter_sche = 0; % schedule iteration
iter_sche2 = 0;

%% 데이터 업데이트 및 check
%duration
for i = 1:size(state,2)
    state(2,i) = state(2,i) + 1; % iteration
    if (state(1,i) == 1) && (state(3,i) ~= 0)
        % schedule update
        if size(sche,1) == 25
            iter_sche = sche(25,i);
            if (state(8,i) ~= 0) && (iter_sche ~= 0)
                % schedule - initial SoC
                %chg
                if (sche(iter_sche,i) >= 0)
                    state(4,i) = round((state(4,i) * state(3,i) + sche(iter_sche,i)*(time_slot/60))*(state(11,i)/100)/state(3,i),2);
                else
                    %dchg
                    state(4,i) = round((state(4,i) * state(3,i) + sche(iter_sche,i)*(time_slot/60))*(state(12,i)/100)/state(3,i),2);
                end
%                 sche(25,i) = sche(25,i) + 1; % schedule iteration update
            end
        end
        % duration
        state(8,i) = state(8,i) - 1;
    end

    % 불확실성 버전도 schedule 적용
    state2(2,i) = state2(2,i) + 1; % iteration
    if (state2(1,i) == 1) && (state2(3,i) ~= 0)
        if size(sche,1) == 25
            iter_sche2 = 0;
            iter_sche2 = sche(25,i);
            if (state2(8,i) ~= 0) && (iter_sche2 ~= 0)
                if (sche(iter_sche2,i) >= 0)
                    state2(4,i) = round((state2(4,i) * state2(3,i) + sche(iter_sche2,i)*(time_slot/60))*(state2(11,i)/100)/state2(3,i),2);
                else
                    state2(4,i) = round((state2(4,i) * state2(3,i) + sche(iter_sche2,i)*(time_slot/60))*(state2(12,i)/100)/state2(3,i),2);
                end
            end
        end
        % duration
        state2(8,i) = state2(8,i) - 1;
    end
end

schedule = zeros(25,size(sche,2));
evse_data = zeros(12,size(evse2,2));
evse_uncert = zeros(12,size(evse2,2));

schedule = sche;
evse_data = state;
evse_uncert = state2;
